simulink model "PD_statespace_practice_d"  (R2020a)
settings: Solver=FixedStepAuto  StartTime=0.0  StopTime=100  FixedStep=Ts  RelTol=1e-3  EnableMultiTasking=on
values from neighbouring files (symbols this model uses):
  down = -up    (= -0.0785398163397)    [PD_statespace.m]
  Kx = place(A_d_x,1.1*B_d_x,p_d_x)    [PD_statespace.m]
  Ky = place(A_d_y,1.1*B_d_y,p_d_y)    [PD_statespace.m]
  Ts = 0.02    [PD_statespace.m]
  up = 4.5*pi/180    (= 0.0785398163397)    [PD_statespace.m]
undefined symbols (not defined in the file or in its folder): DiscIntNeverNeededParam
libraries: raspberrypiBasiclib x6, simulink x3, raspberrypiCommlib x1
settings Model: Creator=hhiastt  LastModifiedBy=hhiastt
settings SolverCC: PositivePriorityOrder=on
settings OptimizationCC: EnhancedBackFolding=on  PassReuseOutputArgsAs=Individual arguments  ZeroExternalMemoryAtStartup=off  ZeroInternalMemoryAtStartup=off  MaxStackSize=64  OptimizeBlockOrder=speed  DifferentSizesBufferReuse=on  OptimizationCustomize=off  EfficientTunableParamExpr=on
settings DebuggingCC: ParameterTunabilityLossMsg=error
settings HardwareCC: ProdBitPerPointer=32  ProdBitPerSizeT=32  ProdBitPerPtrDiffT=32  ProdLargestAtomicInteger=Long  ProdLargestAtomicFloat=Double  ProdWordSize=32  ProdLongLongMode=on  ProdHWDeviceType=ARM Compatible->ARM Cortex
settings RTWCC: SystemTargetFile=ert.tlc  HardwareBoard=Raspberry Pi  TemplateMakefile=ert_default_tmf  Toolchain=GNU GCC Raspberry Pi  BuildConfiguration=Faster Runs
settings CodeAppCC: ForceParamTrailComments=on  IgnoreCustomStorageClasses=off  OperatorAnnotations=on  SimulinkDataObjDesc=on  SFDataObjDesc=on  InsertBlockDesc=on
settings ERTTargetCC: SupportVariableSizeSignals=on

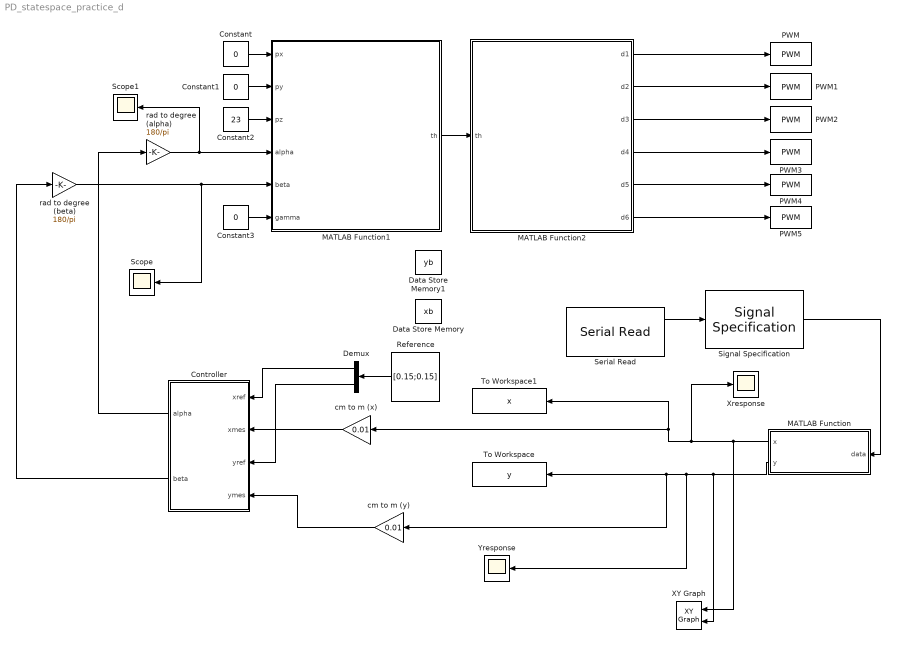
== system PD_statespace_practice_d ==
  Constant : Constant  Value=0
  Constant1 : Constant  Value=0
  Constant2 : Constant  Value=23
  Constant3 : Constant  Value=0
  Controller : Subsystem
  Data Store Memory : DataStoreMemory  DataStoreName=xb  ReadBeforeWriteMsg=warning  WriteAfterWriteMsg=warning  WriteAfterReadMsg=warning  ShowAdditionalParam=off  OutDataTypeStr=double
  Data Store Memory1 : DataStoreMemory  DataStoreName=yb  ReadBeforeWriteMsg=warning  WriteAfterWriteMsg=warning  WriteAfterReadMsg=warning  ShowAdditionalParam=off  OutDataTypeStr=double
  Demux : Demux  Outputs=2
  MATLAB Function : MATLAB Function  TreatAsAtomicUnit=on
  MATLAB Function1 : MATLAB Function  TreatAsAtomicUnit=on
  MATLAB Function2 : MATLAB Function  TreatAsAtomicUnit=on
  PWM : raspberrypiBasiclib/PWM  board=Pi 3 Model B+  Pin_=12  Frequency=50  blockPlatform=Raspberry Pi
      settings: SourceProductBaseCode=RASPPI
  PWM1 : raspberrypiBasiclib/PWM  board=Pi 3 Model B+  Pin_=20  Frequency=50  blockPlatform=Raspberry Pi
      settings: SourceProductBaseCode=RASPPI
  PWM2 : raspberrypiBasiclib/PWM  board=Pi 3 Model B+  Pin_=16  Frequency=50  blockPlatform=Raspberry Pi
      settings: SourceProductBaseCode=RASPPI
  PWM3 : raspberrypiBasiclib/PWM  board=Pi 3 Model B+  Pin_=17  Frequency=50  blockPlatform=Raspberry Pi
      settings: SourceProductBaseCode=RASPPI
  PWM4 : raspberrypiBasiclib/PWM  board=Pi 3 Model B+  Pin_=27  Frequency=50  blockPlatform=Raspberry Pi
      settings: SourceProductBaseCode=RASPPI
  PWM5 : raspberrypiBasiclib/PWM  board=Pi 3 Model B+  Pin_=22  Frequency=50  blockPlatform=Raspberry Pi
      settings: SourceProductBaseCode=RASPPI
  Reference : Constant  Value=[0.15;0.15]
  Scope : Scope
  Scope1 : Scope
  Serial Read : raspberrypiCommlib/Serial Read  board=Pi 3 Model B+  SCIModule_=/dev/ttyS0  Baudrate_=19200  Parity=None  StopBits_=1  HardwareFlowControl=None  ByteOrder=LittleEndian  DataLength=10  DataType=uint8  OutputStatus=on  SampleTime=Ts  blockPlatform=RaspberryPi
      settings: SourceProductBaseCode=RASPPI
  Signal Specification : SignalSpecification  OutDataTypeStr=uint8  Dimensions=10  SampleTime=Ts
  To Workspace : ToWorkspace  VariableName=y  SampleTime=Ts
      settings: Save2DSignal=2-D array (concatenate along first dimension)
  To Workspace1 : ToWorkspace  VariableName=x  SampleTime=Ts
      settings: Save2DSignal=2-D array (concatenate along first dimension)
  XY Graph : simulink/Sinks/XY Graph  xmin=0  xmax=20  ymin=0  ymax=30  st=Ts
  Xresponse : Scope
  Yresponse : Scope
  cm to m (x) : Gain  Gain=0.01
  cm to m (y) : Gain  Gain=0.01
  rad to degree (alpha) : Gain  Gain=180/pi
  rad to degree (beta) : Gain  Gain=180/pi
  wires:
  MATLAB Function2/4(d4) -> PWM3/1
  MATLAB Function2/2(d2) -> PWM1/1
  Constant2/1 -> MATLAB Function1/3(pz)
  Signal Specification/1 -> MATLAB Function/1(data)
  MATLAB Function2/3(d3) -> PWM2/1
  MATLAB Function2/6(d6) -> PWM5/1
  Constant1/1 -> MATLAB Function1/2(py)
  MATLAB Function/2(y) -> XY Graph/2, cm to m (y)/1, To Workspace/1, Yresponse/1
  Serial Read/1 -> Signal Specification/1
  rad to degree (beta)/1 -> MATLAB Function1/5(beta), Scope/1
  rad to degree (alpha)/1 -> Scope1/1, MATLAB Function1/4(alpha)
  MATLAB Function/1(x) -> Xresponse/1, To Workspace1/1, cm to m (x)/1, XY Graph/1
  MATLAB Function2/5(d5) -> PWM4/1
  Controller/1(alpha) -> rad to degree (alpha)/1
  cm to m (x)/1 -> Controller/2(xmes)
  Constant/1 -> MATLAB Function1/1(px)
  MATLAB Function1/1(th) -> MATLAB Function2/1(th)
  MATLAB Function2/1(d1) -> PWM/1
  cm to m (y)/1 -> Controller/4(ymes)
  Controller/2(beta) -> rad to degree (beta)/1
  Reference/1 -> Demux/1
  Demux/2 -> Controller/3(yref)
  Demux/1 -> Controller/1(xref)
  Constant3/1 -> MATLAB Function1/6(gamma)

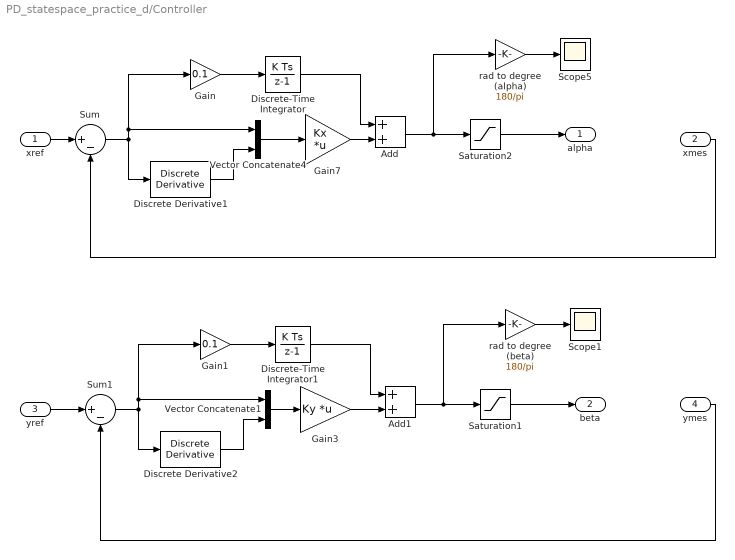
== system PD_statespace_practice_d/Controller ==
  xref : Inport
  xmes : Inport  Port=2
  yref : Inport  Port=3
  ymes : Inport  Port=4
  Add : Sum
  Add1 : Sum
  Discrete Derivative1 : simulink/Discrete/Discrete Derivative  gainval=1.0  ICPrevScaledInput=0.0  OutMin=[]  OutMax=[]  OutDataType=fixdt(1, 16)  OutScaling=2^-10  DoSatur=off
  Discrete Derivative2 : simulink/Discrete/Discrete Derivative  gainval=1.0  ICPrevScaledInput=0.0  OutMin=[]  OutMax=[]  OutDataType=fixdt(1, 16)  OutScaling=2^-10  DoSatur=off
  Discrete-Time Integrator : DiscreteIntegrator  SampleTime=-1  ICPrevOutput=DiscIntNeverNeededParam  ICPrevScaledInput=DiscIntNeverNeededParam
  Discrete-Time Integrator1 : DiscreteIntegrator  SampleTime=-1  ICPrevOutput=DiscIntNeverNeededParam  ICPrevScaledInput=DiscIntNeverNeededParam
  Gain : Gain  Gain=0.1
  Gain1 : Gain  Gain=0.1
  Gain3 : Gain  Gain=Ky  Multiplication=Matrix(K*u)
  Gain7 : Gain  Gain=Kx  Multiplication=Matrix(K*u)
  Saturation1 : Saturate  UpperLimit=up  LowerLimit=down
  Saturation2 : Saturate  UpperLimit=up  LowerLimit=down
  Scope1 : Scope
  Scope5 : Scope
  Sum : Sum  Inputs=|+-
  Sum1 : Sum  Inputs=|+-
  Vector Concatenate1 : Concatenate
  Vector Concatenate4 : Concatenate
  rad to degree (alpha) : Gain  Gain=180/pi
  rad to degree (beta) : Gain  Gain=180/pi
  alpha : Outport
  beta : Outport  Port=2
  wires:
  xref/1 -> Sum/1
  Saturation2/1 -> alpha/1
  rad to degree (alpha)/1 -> Scope5/1
  xmes/1 -> Sum/2
  Sum/1 -> Vector Concatenate4/1, Gain/1, Discrete Derivative1/1
  Vector Concatenate4/1 -> Gain7/1
  Discrete Derivative1/1 -> Vector Concatenate4/2
  Gain7/1 -> Add/2
  Add/1 -> rad to degree (alpha)/1, Saturation2/1
  Discrete-Time Integrator/1 -> Add/1
  Gain/1 -> Discrete-Time Integrator/1
  Gain1/1 -> Discrete-Time Integrator1/1
  Discrete-Time Integrator1/1 -> Add1/1
  Add1/1 -> rad to degree (beta)/1, Saturation1/1
  Gain3/1 -> Add1/2
  ymes/1 -> Sum1/2
  Saturation1/1 -> beta/1
  Sum1/1 -> Vector Concatenate1/1, Gain1/1, Discrete Derivative2/1
  rad to degree (beta)/1 -> Scope1/1
  Vector Concatenate1/1 -> Gain3/1
  Discrete Derivative2/1 -> Vector Concatenate1/2
  yref/1 -> Sum1/1

== matlab function PD_statespace_practice_d/MATLAB Function1 ==
  data: px input double size=1; th output double; py input double size=1; pz input double size=1; alpha input double size=1; beta input double size=1; gamma input double size=1
function th = inv_ken_test(px,py,pz,alpha,beta,gamma)
th=zeros(1,6);
l1=3.2;
l2=25.57;
b=26;
d=20;
b1=30;
d1=6;
RA1=[(1/sqrt(12))*(2*b+d);d/2;0];
RA2=[-(1/sqrt(12))*(b-d);(b+d)/2;0];
RA3=[-(1/sqrt(12))*(b+2*d);b/2;0];
RA4=[-(1/sqrt(12))*(b+2*d);-b/2;0];
RA5=[-(1/sqrt(12))*(b-d);-(b+d)/2;0];
RA6=[(1/sqrt(12))*(2*b+d);-d/2;0];
RA=[RA1 RA2 RA3 RA4 RA5 RA6];

RC1=[(1/sqrt(12))*(b1+2*d1);b1/2;0];
RC2=[(1/sqrt(12))*(b1-d1);(b1+d1)/2;0];
RC3=[-(1/sqrt(12))*(2*b1+d1);d1/2;0];
RC4=[-(1/sqrt(12))*(2*b1+d1);-d1/2;0];
RC5=[(1/sqrt(12))*(b1-d1);-(b1+d1)/2;0];
RC6=[(1/sqrt(12))*(b1+2*d1);-b1/2;0];
RC=[RC1 RC2 RC3 RC4 RC5 RC6];

v=[0 0 0 1];
T_base_A1=[rotz(150)*rotx(90) RA1;v];
T_base_A2=[rotz(-30)*rotx(90) RA2;v];
T_base_A3=[rotz(-90)*rotx(90) RA3;v];
T_base_A4=[rotz(90)*rotx(90) RA4;v];
T_base_A5=[rotz(30)*rotx(90) RA5;v];
T_base_A6=[rotz(-150)*rotx(90) RA6;v];

% Computation
R=[rotz(gamma)*roty(beta)*rotx(alpha);0 0 0];
P=[px;py;pz;1];
T=[R P];
RCE=T*[RC;ones(1,6)];
RAE=[RA;ones(1,6)];
L=zeros(1,6);
for i =1:6
    L(i)=sum((RCE(:,i)-RAE(:,i)).^2)^0.5;
end

RA1C1=T_base_A1^(-1)*(RCE(:,1)-RAE(:,1));
RA2C2=T_base_A2^(-1)*(RCE(:,2)-RAE(:,2));
RA3C3=T_base_A3^(-1)*(RCE(:,3)-RAE(:,3));
RA4C4=T_base_A4^(-1)*(RCE(:,4)-RAE(:,4));
RA5C5=T_base_A5^(-1)*(RCE(:,5)-RAE(:,5));
RA6C6=T_base_A6^(-1)*(RCE(:,6)-RAE(:,6));
RAC=[RA1C1 RA2C2 RA3C3 RA4C4 RA5C5 RA6C6];
P1=zeros(1,6);
G1=zeros(1,6);
for i=1:6
    P1(i)=(L(i)^2+l1^2-l2^2)/(2*l1);
end
for i=1:6
    G1(i)=RAC(1,i)^2+RAC(2,i)^2-(P1(i)^2);
end
delta=1;
for i=1:6
    th(i)=atan2d(P1(i)*RAC(2,i)+RAC(1,i)*delta*sqrt(G1(i)), ...
        abs(P1(i)*RAC(1,i)-RAC(2,i)*delta*sqrt(G1(i))));
end

== matlab function PD_statespace_practice_d/MATLAB Function ==
  data: data input; x output; y output; xb data_store_memory; yb data_store_memory
function [x,y] = process_data(data)
global xb
global yb
x=0;y=0;xx=0;yy=0;j=0;data1=zeros(1,4);
data2=zeros(1,4);
for i=1:10
    if(data(i) == 255)
        j=i;
    end
end
if(j <= 6 && j>0)
    data1=data(j+1:j+4);
    data2=cast(data1,'like',zeros(1,4));    
    xx=data2(1)*256+data2(2);
    yy=data2(3)*256+data2(4);
    xx=(xx-floor(floor(xx/128)/2)*128)/2;
    yy=(yy-floor(floor(yy/128)/2)*128)/2;
    x=((xx-20)/470)*22.8;
    y=((yy-7)/490)*30.4;
    xb=x;
    yb=y;
else
    x=xb;
    y=yb;
end
end

== matlab function PD_statespace_practice_d/MATLAB Function2 ==
  data: th input double size=6; d1 output double size=1; d2 output; d3 output; d4 output; d5 output; d6 output
function [d1,d2,d3,d4,d5,d6] =    Angle2duty_test(th)
M1=[0,1.14;10,1.23;20,1.29;30,1.38;40,1.45;50,1.53;60,1.61];
p1=polyfit(M1(:,1),M1(:,2),1);
M2=[0,1.67;10,1.76;20,1.83;30,1.91;40,2];
p2=polyfit(M2(:,1),M2(:,2),1);
M3=[0,1.24;10,1.33;20,1.42;30,1.49;40,1.56;50,1.64];
p3=polyfit(M3(:,1),M3(:,2),1);
M4=[0,1.68;10,1.75;20,1.84;30,1.92;37,1.99];
p4=polyfit(M4(:,1),M4(:,2),1);
M5=[0,1.14;10,1.22;20,1.3;30,1.37;40,1.45;50,1.53];
p5=polyfit(M5(:,1),M5(:,2),1);
M6=[0,1.68;10,1.75;20,1.84;26,1.86];
p6=polyfit(M6(:,1),M6(:,2),1);
d=zeros(1,6);
d1=dot(p1,[th(1),1])/20;
d2=dot(p2,[-th(2),1])/20;
d3=dot(p3,[th(3),1])/20;
d4=dot(p4,[-th(4),1])/20;
d5=dot(p5,[th(5),1])/20;
d6=dot(p6,[-th(6),1])/20;
